simulink model "ModelCfact40"  (R2018a)
settings: Solver=ode23  StartTime=0.0  StopTime=0.1  MaxStep=10e-6  RelTol=1e-3
libraries: powerlib x17
settings Model: Creator=ivank  LastModifiedBy=bw_
settings SolverCC: InitialStep=10e-8

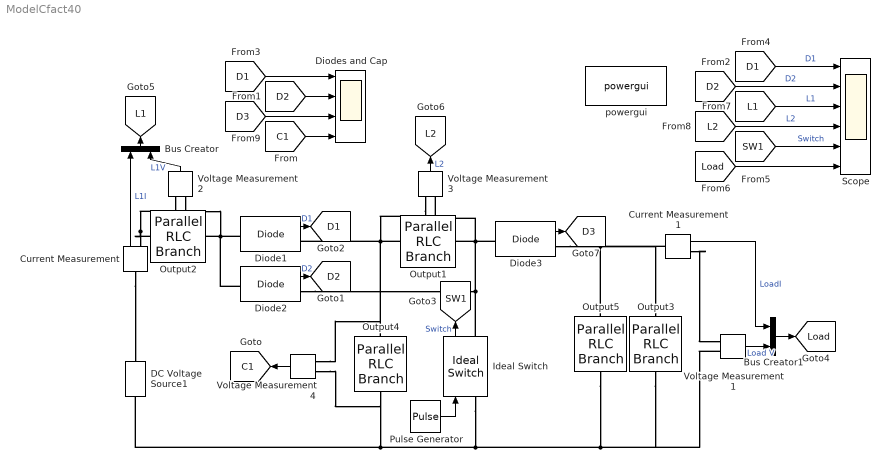
== system ModelCfact40 ==
  Bus Creator : BusCreator  Inputs=2
  Bus Creator1 : BusCreator  Inputs=2
  Current Measurement : powerlib/Measurements/Current Measurement  PhasorSimulation=off  OutputType=Complex  PSBequivalent=0
  Current Measurement1 : powerlib/Measurements/Current Measurement  PhasorSimulation=off  OutputType=Complex  PSBequivalent=0
  DC Voltage Source1 : powerlib/Electrical Sources/DC Voltage Source  Amplitude=10  Measurements=None
  Diode1 : powerlib/Power Electronics/Diode  Ron=0.001  Lon=0  Vf=0.8  IC=0  UseSnubber=0  Rs=500  Cs=250e-9  Measurements=on
  Diode2 : powerlib/Power Electronics/Diode  Ron=0.001  Lon=0  Vf=0.8  IC=0  UseSnubber=0  Rs=500  Cs=250e-9  Measurements=on
  Diode3 : powerlib/Power Electronics/Diode  Ron=0.001  Lon=0  Vf=0.8  IC=0  UseSnubber=0  Rs=500  Cs=250e-9  Measurements=on
  Diodes and Cap : Scope  NumInputPorts=4
  Ideal Switch : powerlib/Power Electronics/Ideal Switch  Ron=0.001  Lon=0  IC=0  Rs=1e5  Cs=inf  Measurements=on
  Output1 : powerlib/Elements/Parallel RLC Branch  LConnTagsString=a  RConnTagsString=__new0  BranchType=L  Resistance=7.225  Inductance=150e-6  SetiL0=off  InitialCurrent=0  Capacitance=100*10e-6  Setx0=off  InitialVoltage=0  Measurements=Branch voltage and current
  Output2 : powerlib/Elements/Parallel RLC Branch  LConnTagsString=a  RConnTagsString=__new0  BranchType=L  Resistance=7.225  Inductance=150e-6  SetiL0=off  InitialCurrent=0  Capacitance=100*10e-6  Setx0=off  InitialVoltage=0  Measurements=Branch voltage and current
  Output3 : powerlib/Elements/Parallel RLC Branch  LConnTagsString=a  RConnTagsString=__new0  BranchType=R  Resistance=225  Inductance=1e-3  SetiL0=off  InitialCurrent=0  Capacitance=100*10e-6  Setx0=off  InitialVoltage=0  Measurements=Branch voltage and current
  Output4 : powerlib/Elements/Parallel RLC Branch  LConnTagsString=a  RConnTagsString=__new0  BranchType=C  Resistance=7.225  Inductance=1e-3  SetiL0=off  InitialCurrent=0  Capacitance=220e-6  Setx0=off  InitialVoltage=0  Measurements=Branch voltage and current
  Output5 : powerlib/Elements/Parallel RLC Branch  LConnTagsString=a  RConnTagsString=__new0  BranchType=C  Resistance=7.225  Inductance=1e-3  SetiL0=off  InitialCurrent=0  Capacitance=220e-6  Setx0=off  InitialVoltage=0  Measurements=Branch voltage and current
  Pulse Generator : DiscretePulseGenerator  PulseType=Time based  Period=1/1000  PulseWidth=50
  Scope : Scope  NumInputPorts=6
  Voltage Measurement{1..4} (4 alike) : powerlib/Measurements/Voltage Measurement  PhasorSimulation=off  OutputType=Complex  PSBequivalent=0
  powergui : powerlib/powergui  Priority=1  SimulationMode=Continuous  SampleTime=50e-6  frequency=60  Iterations=50  frequencyindice=0  Pbase=100e6  ErrMax=1e-4  UnitsV=kV  UnitsW=MW  buscounter=0  FunctionMessages=off  echomessages=off  EnableUseOfTLC=off  CurrentSourceSwitches=off  DisableSnubberDevices=off  DisableRonSwitches=off  DisableVfSwitches=off  DisplayEquations=off  SolverType=Tustin/Backward Euler (TBE)  Interpol=off  ExternalGateDelay=off  methode=off  Ts=100  x0status=blocks  SPID=on  SwTol=0  HookPort=off  RestoreLinks=warning  ResistiveCurrentMeasurement=off  Frange=[0:2:500]  Ylog=off  Xlog=on  ShowGrid=off  save=off  variable=ZData  structure=0  ZoomFFT=off  StartTime=0.0  cycles=1  DisplayStyle=1  fundamental=60  FreqAxis=off  MaxFrequency=1000  frequencyindicesteady=1  RmsSteady=1  display=off
  tag scope: C1=global, D1=global, D2=global, D3=global, L1=global, L2=global, Load=global, SW1=global
  wires:
  [Load] -> Scope/6
  Pulse Generator/1 -> Ideal Switch/1
  [L1] -> Scope/3  "L1"
  [L2] -> Scope/4  "L2"
  [SW1] -> Scope/5  "Switch"
  Voltage Measurement4/1 -> [C1]
  [C1] -> Diodes and Cap/4
  Diode2/1 -> [D2]  "D2"
  [D2] -> Diodes and Cap/2
  [D2] -> Scope/2  "D2"
  Diode1/1 -> [D1]  "D1"
  [D1] -> Diodes and Cap/1
  [D1] -> Scope/1  "D1"
  Ideal Switch/1 -> [SW1]  "Switch"
  Voltage Measurement1/1 -> Bus Creator1/2  "Load V"
  Voltage Measurement2/1 -> Bus Creator/2  "L1V"
  Voltage Measurement3/1 -> [L2]  "L2"
  Diode3/1 -> [D3]
  [D3] -> Diodes and Cap/3
  Current Measurement/1 -> Bus Creator/1  "L1I"
  Bus Creator/1 -> [L1]
  Current Measurement1/1 -> Bus Creator1/1  "LoadI"
  Bus Creator1/1 -> [Load]
  connections:
  Ideal Switch/LConn1 -- Voltage Measurement1/LConn2 -- Output3/RConn1 -- Output5/RConn1 -- Voltage Measurement4/LConn2 -- Output4/RConn1 -- DC Voltage Source1/LConn1
  Output2/RConn1 -- Voltage Measurement2/LConn2 -- Current Measurement/RConn1
  Diode1/LConn1 -- Diode2/LConn1 -- Voltage Measurement2/LConn1 -- Output2/LConn1
  Output1/RConn1 -- Voltage Measurement4/LConn1 -- Output4/LConn1 -- Diode1/RConn1 -- Voltage Measurement3/LConn2
  Ideal Switch/RConn1 -- Diode2/RConn1 -- Diode3/LConn1 -- Voltage Measurement3/LConn1 -- Output1/LConn1
  Output3/LConn1 -- Current Measurement1/LConn1 -- Output5/LConn1 -- Diode3/RConn1
  Current Measurement/LConn1 -- DC Voltage Source1/RConn1
  Current Measurement1/RConn1 -- Voltage Measurement1/LConn1
